simulink library "VLS"  (R2022b)
settings: Solver=VariableStepAuto  StartTime=0.0  StopTime=10.0  RelTol=1e-3
undefined symbols (not defined in the file or in its folder): repelem, VLSConfig
libraries: dspmtrx3 x2, FeaturePath x2, VLSGen x2, XtalkCancellation x1
settings Model: Creator=ud1041536  LastModifiedBy=mt1047270
settings SolverCC: AlgebraicLoopSolver=TrustRegion
settings DebuggingCC: UnconnectedInputMsg=warning  UnconnectedOutputMsg=warning  UnconnectedLineMsg=warning  SFMachineParentedDataDiag=warning
settings ModelReferenceCC: EnableRefExpFcnMdlSchedulingChecks=on

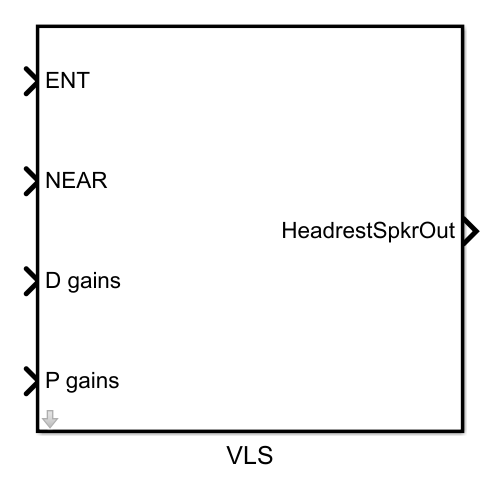
[thumbnail: Simulink's stored preview of the top-level diagram]
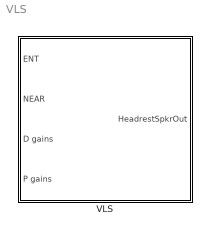
== system VLS ==
  VLS : Subsystem  TreatAsAtomicUnit=on  mask(Virtual Loudspeaker){configStruct=VLSConfig}
      mask prompts: configStruct "Config struct name:"
      mask init:
      | numGains = configStruct.VLSGainsConfig.numGains;
      settings: RTWSystemCode=Nonreusable function  RTWFcnNameOpts=Use subsystem name  RTWFileNameOpts=Use subsystem name  FunctionWithSeparateData=on

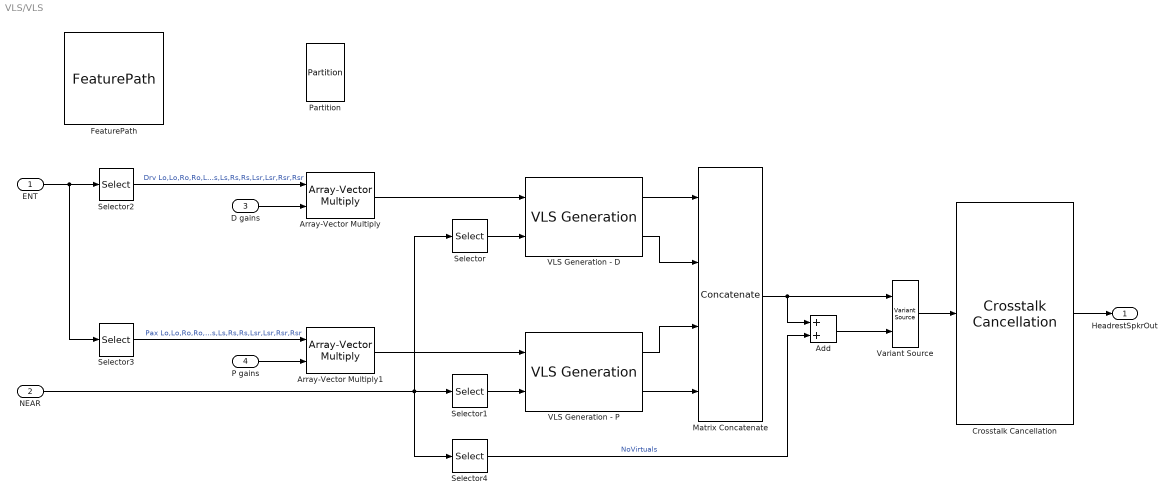
== system VLS/VLS ==
  ENT : Inport
  NEAR : Inport  Port=2
  D gains : Inport  Port=3
  P gains : Inport  Port=4
  Add : Sum
  Array-Vector Multiply : dspmtrx3/Array-Vector Multiply  mode=Mute  saveAsFlag=0  Dimension=2  V_Source=Input port  V_VectFromMask=[0.5 0.25]  roundingMode=Floor  overflowMode=off  firstCoeffSignedness=Auto  firstCoeffDataTypeStr=Inherit: Same word length as input  firstCoeffMin=[]  firstCoeffMax=[]  firstCoeffLastDataTypeStr=Inherit: Same word length as input  prodOutputSignedness=Auto  accumSignedness=Auto  outputSignedness=Auto  outputDataTypeStr=Inherit: Same as product output  outputMin=[]  outputMax=[]  outputLastDataTypeStr=Inherit: Same as product output
  Array-Vector Multiply1 : dspmtrx3/Array-Vector Multiply  mode=Mute  saveAsFlag=0  Dimension=2  V_Source=Input port  V_VectFromMask=[0.5 0.25]  roundingMode=Floor  overflowMode=off  firstCoeffSignedness=Auto  firstCoeffDataTypeStr=Inherit: Same word length as input  firstCoeffMin=[]  firstCoeffMax=[]  firstCoeffLastDataTypeStr=Inherit: Same word length as input  prodOutputSignedness=Auto  accumSignedness=Auto  outputSignedness=Auto  outputDataTypeStr=Inherit: Same as product output  outputMin=[]  outputMax=[]  outputLastDataTypeStr=Inherit: Same as product output
  Crosstalk Cancellation : XtalkCancellation/Crosstalk Cancellation  configStruct=configStruct.XtalkCancellationConfig
  FeaturePath : FeaturePath/FeaturePath  FeatureName=VLS  IsGroup=off  GroupNumber=-1  IsModule=off  TriggerInit=[1295 -226 1410 -119]
      settings: SourceProductName=Bose Talaria
  Matrix Concatenate : Concatenate  NumInputs=4  Mode=Multidimensional array  ConcatenateDimension=2
  Partition : FeaturePath/Partition  PartitionNumber=0  TriggerInit=[1575 -214 1620 -146]
      settings: SourceProductName=Bose Talaria
  Selector : Selector  NumberOfDimensions=2  InputPortWidth=3  IndexOptions=Select all,Index vector (dialog)  Indices=[1 3],1:numGains  OutputSizes=1,1
  Selector1 : Selector  NumberOfDimensions=2  InputPortWidth=3  IndexOptions=Select all,Index vector (dialog)  Indices=[1 3],numGains + (1:numGains)  OutputSizes=1,1
  Selector2 : Selector  NumberOfDimensions=2  InputPortWidth=3  IndexOptions=Select all,Index vector (dialog)  Indices=[1 3],repelem(1:6,2)  OutputSizes=1,1
  Selector3 : Selector  NumberOfDimensions=2  InputPortWidth=3  IndexOptions=Select all,Index vector (dialog)  Indices=[1 3],repelem(7:12,2)  OutputSizes=1,1
  Selector4 : Selector  NumberOfDimensions=2  InputPortWidth=3  IndexOptions=Select all,Starting index (dialog)  Indices=[1 3],numGains*2+1  OutputSizes=1,4
  VLS Generation - D : VLSGen/VLS Generation  configStruct=configStruct.VLSGenDConfig  FeatureName=GenerationDrv
  VLS Generation - P : VLSGen/VLS Generation  configStruct=configStruct.VLSGenPConfig  FeatureName=GenerationPax
  Variant Source : VariantSource
  HeadrestSpkrOut : Outport
  wires:
  Crosstalk Cancellation/1 -> HeadrestSpkrOut/1
  Selector/1 -> VLS Generation - D/2
  P gains/1 -> Array-Vector Multiply1/2
  Selector1/1 -> VLS Generation - P/2
  ENT/1 -> Selector3/1, Selector2/1
  Array-Vector Multiply1/1 -> VLS Generation - P/1
  Array-Vector Multiply/1 -> VLS Generation - D/1
  NEAR/1 -> Selector4/1, Selector/1, Selector1/1
  Selector3/1 -> Array-Vector Multiply1/1  "Pax Lo,Lo,Ro,Ro,Ls,Ls,Rs,Rs,Lsr,Lsr,Rsr,Rsr"
  D gains/1 -> Array-Vector Multiply/2
  Selector2/1 -> Array-Vector Multiply/1  "Drv Lo,Lo,Ro,Ro,Ls,Ls,Rs,Rs,Lsr,Lsr,Rsr,Rsr"
  VLS Generation - D/1 -> Matrix Concatenate/1
  VLS Generation - P/2 -> Matrix Concatenate/4
  VLS Generation - P/1 -> Matrix Concatenate/3
  VLS Generation - D/2 -> Matrix Concatenate/2
  Matrix Concatenate/1 -> Variant Source/1, Add/1
  Add/1 -> Variant Source/2
  Selector4/1 -> Add/2  "NoVirtuals"
  Variant Source/1 -> Crosstalk Cancellation/1
